simulink library "Pump_Const"  (Simulink 8.2)
settings: Solver=ode45  StartTime=0.0  StopTime=10.0  RelTol=1e-3
libraries: carnot x2
settings Model: Creator=lena.frank  LastModifiedBy=drhf

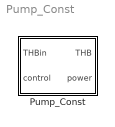
== system Pump_Const ==
  Pump_Const : Subsystem  mask(constant pump){mdotmax=1200/3600, dia=0.0157, power=30, p0=3e5, fluid_id=Water, mix=0, UA=3, mcp=4000, tamb=20}
      mask prompts: mdotmax "massflow rate [kg/s]"; dia "diameter at in- and outlet [m]"; power "electric power consumption [W]"; p0 "system pressure in Pa"; fluid_id "fluid"; mix "percentage of fluid mix [0..1]"; UA "losses to ambient in W/K"; mcp "thermal capacity in J/K"; tamb "ambient temperatature in °C"
      mask help:
      | Set constant massflow rate according to the control signal.
      | The pump has a thermal capacity and losses to ambient.
      mask Help: web(fullfile(path_carnot('help'),'Pump_Const.html'),'-helpbrowser')
      mask TypeOptions fluid_id: Water | Air | Cotton Oil | Silicone Oil | Water-Glycol Mix | Tyfocor LS | Water (Constant 20°C) | Air (dry+ constant 20°C)
      mask Display:
      | plot(0,0,100,100,[40,70,40,30,30,40,60,70,70,60,40],[70,50,30,40,60,70,70,60,40,30,30])
      | port_label('input',1,'THB')
      | port_label('input',2,'ctr')
      | port_label('output',1,'THB')
      | port_label('output',2,'Pel')

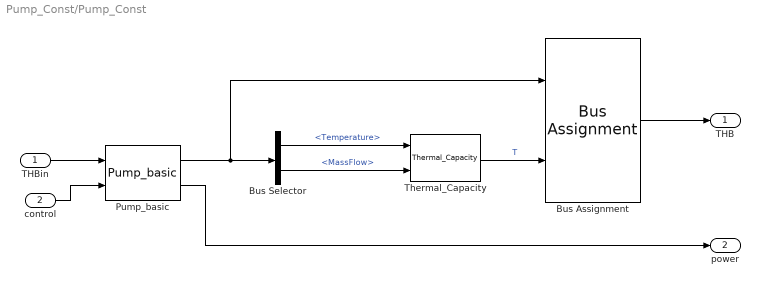
== system Pump_Const/Pump_Const ==
  THBin : Inport
  control : Inport  Port=2
  Bus Assignment : BusAssignment  AssignedSignals=Temperature
  Bus Selector : BusSelector  OutputSignals=Temperature,MassFlow
  Pump_basic : carnot/Basic/Hydraulics/Pump_basic  mdotmax=mdotmax  fluid_id=fluid_id  mix=mix  dia=dia  power=power  p0=p0  hgt=0  ID=1
  Thermal_Capacity : carnot/Basic/Thermal_Models/Thermal_Capacity  UA=UA  mcp=mcp  Tamb=tamb
  THB : Outport
  power : Outport  Port=2
  wires:
  Bus Assignment/1 -> THB/1
  Pump_basic/2 -> power/1
  Bus Selector/2 -> Thermal_Capacity/2  "<MassFlow>"
  control/1 -> Pump_basic/2
  Thermal_Capacity/1 -> Bus Assignment/2  "T"
  Bus Selector/1 -> Thermal_Capacity/1  "<Temperature>"
  THBin/1 -> Pump_basic/1
  Pump_basic/1 -> Bus Selector/1, Bus Assignment/1
